simulink model "motor_DC_"  (R2012a)
settings: Solver=ode45  SolverMode=SingleTasking  StartTime=0.0  StopTime=10.0  RelTol=1e-3
values from neighbouring files (symbols this model uses):
  b = 100000    [ejercicio7_taller2SM.m]    (also in motord_DC_rot.m = 0.1)
  J = 12    [ejercicio7_taller2SM.m]    (also in motord_DC_rot.m = 0.01)
  Kb = 5    [motord_DC_rot.m]
  Kp = 5    [motord_DC_rot.m]
  L = 1e-3    (= 0.001)    [anexo_parcial.m]    (also in ejemplo_electrico.m = 0.1; motord_DC_rot.m = 0.0001)
  R = 10    [anexo_parcial.m]    (also in ejemplo_electrico.m = 1000; ejercicio7_taller2SM.m = 0.01; motord_DC_rot.m; nivel_tanque.m = 37)
settings Model: CovMetricSettings=dwe  CovHtmlReporting=off  covSaveCumulativeToWorkspaceVar=off  CovSaveSingleToWorkspaceVar=off  CovExternalEMLEnable=on  Creator=carma  LastModifiedBy=carma
settings DataIOCC: SaveFormat=StructureWithTime  ReturnWorkspaceOutputs=off
settings OptimizationCC: LifeSpan=inf  SimCompilerOptimization=Off
settings DebuggingCC: FcnCallInpInsideContextMsg=Enable All
settings HardwareCC: ProdWordSize=32  ProdHWDeviceType=Specified
settings SFSimCC: SimUseLocalCustomCode=off
settings RTWCC: RTWUseLocalCustomCode=off  RTWCompilerOptimization=Off
settings GRTTargetCC: CodeReplacementLibrary=C99 (ISO)  CPPClassGenCompliant=off

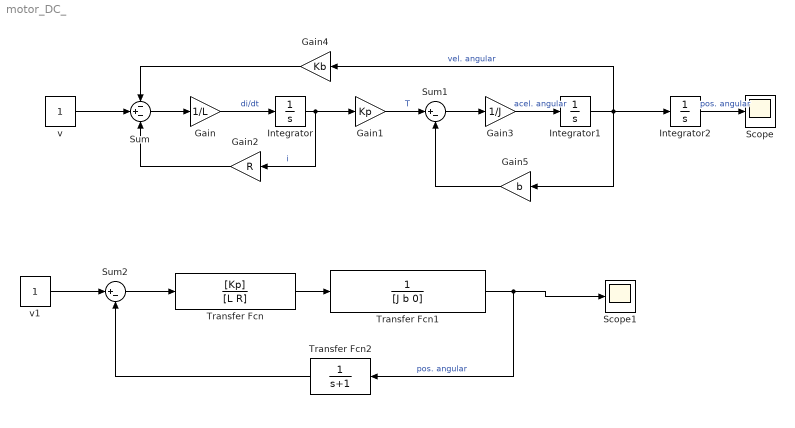
== system motor_DC_ ==
  Gain : Gain  Gain=1/L
  Gain1 : Gain  Gain=Kp
  Gain2 : Gain  Gain=R
  Gain3 : Gain  Gain=1/J
  Gain4 : Gain  Gain=Kb
  Gain5 : Gain  Gain=b
  Integrator : Integrator
  Integrator1 : Integrator
  Integrator2 : Integrator
  Scope : Scope
      settings: TimeRange=auto  MaxDataPoints=5000  SaveToWorkspace=off  SaveName=ScopeData  YMin=-10  YMax=10  SampleTime=-1
  Scope1 : Scope
      settings: TimeRange=auto  MaxDataPoints=5000  SaveToWorkspace=off  YMin=-10  YMax=10  SampleTime=-1
  Sum : Sum  Inputs=-+-
  Sum1 : Sum  Inputs=|+-
  Sum2 : Sum  Inputs=|+-
  Transfer Fcn : TransferFcn  Numerator=[Kp]  Denominator=[L R]
  Transfer Fcn1 : TransferFcn  Denominator=[J b 0]
  Transfer Fcn2 : TransferFcn  Denominator=[1 1]
  v : Constant
  v1 : Constant
  wires:
  v/1 -> Sum/2
  Sum/1 -> Gain/1
  Gain/1 -> Integrator/1  "di/dt"
  Integrator/1 -> Gain2/1, Gain1/1  "i"
  Gain2/1 -> Sum/3
  Gain1/1 -> Sum1/1  "T"
  Sum1/1 -> Gain3/1
  Gain3/1 -> Integrator1/1  "acel. angular"
  Integrator1/1 -> Gain4/1, Gain5/1, Integrator2/1  "vel. angular"
  Integrator2/1 -> Scope/1  "pos. angular"
  Gain5/1 -> Sum1/2
  Gain4/1 -> Sum/1
  Transfer Fcn1/1 -> Transfer Fcn2/1, Scope1/1  "pos. angular"
  Sum2/1 -> Transfer Fcn/1
  Transfer Fcn/1 -> Transfer Fcn1/1
  Transfer Fcn2/1 -> Sum2/2
  v1/1 -> Sum2/1
